simulink model "Understanding_Control_Systems_3"  (R2016b)
settings: Solver=VariableStepAuto  StartTime=0.0  StopTime=400  RelTol=1e-3
PreLoadFcn:
  | Car=Simulink.Variant('vehicleType==1')
  | SportsCar=Simulink.Variant('vehicleType==2')
  | Truck=Simulink.Variant('vehicleType==3')
  | 
  | vehicleType=1
libraries: MeldasLibrary x5, simulink x1
settings Model: Creator=mulusoy  LastModifiedBy=mulusoy
settings DebuggingCC: SFUnconditionalPathOutOfParentDiag=warning  SFUnreachableStateOrJunctionDiag=warning  SFDanglingTransitionDiag=warning
settings CodeAppCC: CustomSymbolStrSimulinkFcn=$N
settings ConfigComp: CovMetricSettings=dswe

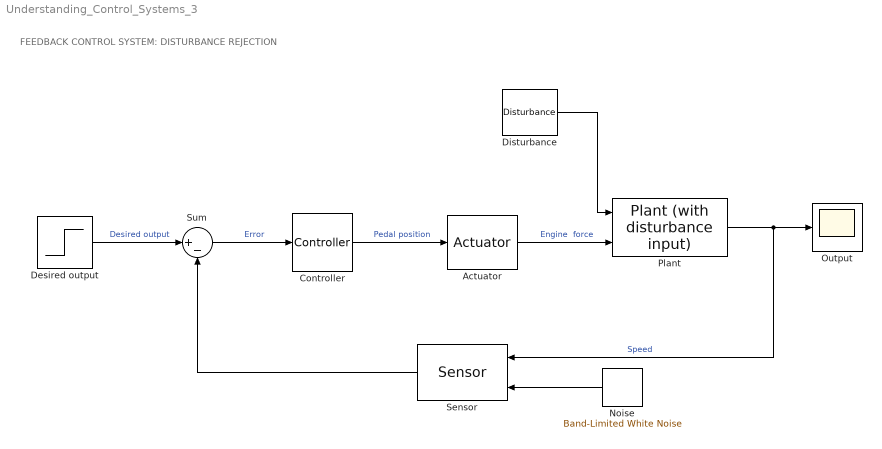
== system Understanding_Control_Systems_3 ==
  note: FEEDBACK CONTROL SYSTEM: DISTURBANCE REJECTION
  Actuator : MeldasLibrary/Actuator  SystemSampleTime=-1
  Controller : MeldasLibrary/Controller  SystemSampleTime=-1
  Desired output : Step  Time=5  After=20  SampleTime=0
  Disturbance : MeldasLibrary/Disturbance  SystemSampleTime=-1
  Noise : simulink/Sources/Band-Limited White Noise  Cov=0.01  Ts=0.1  seed=[23341]
  Output : Scope
  Plant : MeldasLibrary/Plant (with disturbance input)  vehicleType=Car
  Sensor : MeldasLibrary/Sensor  SystemSampleTime=-1
  Sum : Sum  Inputs=|+-
  wires:
  Controller/1 -> Actuator/1  "Pedal position"
  Actuator/1 -> Plant/2  "Engine  force"
  Plant/1 -> Sensor/1, Output/1  "Speed"
  Disturbance/1 -> Plant/1
  Noise/1 -> Sensor/2
  Desired output/1 -> Sum/1  "Desired output"
  Sensor/1 -> Sum/2
  Sum/1 -> Controller/1  "Error"
